simulink model "untitled"  (R2023b)
settings: Solver=VariableStepAuto  StartTime=0.0  StopTime=10  RelTol=1e-3
values from neighbouring files (symbols this model uses):
  A = [0, 1, 0, 0, 0, 0 ... (first row only)    [DESACOPLE.m]    (also in untitled2.m = (subs(A_sym, [qs; fs], [qs0; fs0])))
  B = [0, 0, 0; 50/(25*q3_op^2 +10*q3_op +3), 0, 0;0, 0, 0;0, 2/3, 0;0, 0, 0;0, 0, 2]    [DESACOPLE.m]    (also in untitled2.m = (subs(B_sym, [qs; fs], [qs0; fs0])))
  F = G*P    [DESACOPLE.m]
  G = pinv(E)    [DESACOPLE.m]
  q3_op = 0.2    [DESACOPLE.m]
undefined symbols (not defined in the file or in its folder): A_num, B_num
settings Model: Creator=alejo  LastModifiedBy=alejo

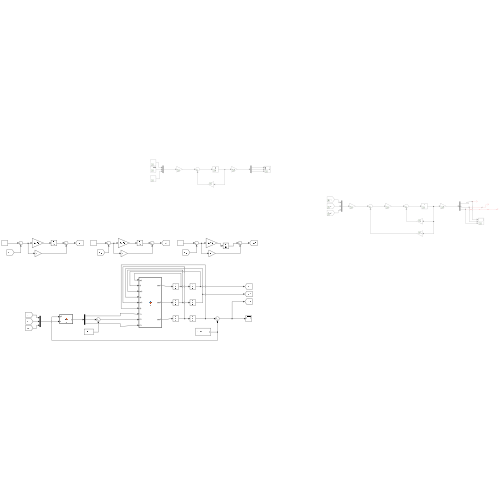
[thumbnail: Simulink's stored preview of the top-level diagram]
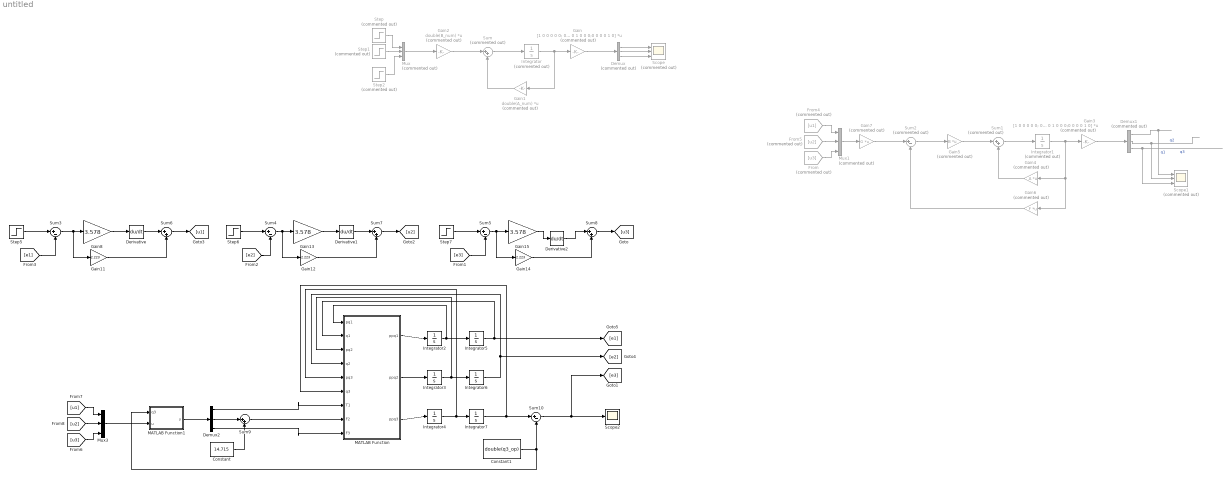
== system untitled ==
  Constant : Constant  Value=14.715
  Constant1 : Constant  Value=double(q3_op)
  Demux : Demux  Commented=on  Outputs=3
  Demux1 : Demux  Commented=on  Outputs=3
  Demux2 : Demux  Outputs=3
  Derivative : Derivative
  Derivative1 : Derivative
  Derivative2 : Derivative
  From : From  Commented=on  GotoTag=u3
  From4 : From  Commented=on  GotoTag=u1
  From5 : From  Commented=on  GotoTag=u2
  Gain : Gain  Commented=on  Gain=[1 0 0 0 0 0; 0 0 1 0 0 0;0 0 0 0 1 0]  Multiplication=Matrix(K*u)
  Gain1 : Gain  Commented=on  Gain=double(A_num)  Multiplication=Matrix(K*u)
  Gain11 : Gain  Gain=2.223
  Gain12 : Gain  Gain=2.223
  Gain13 : Gain  Gain=3.578
  Gain14 : Gain  Gain=2.223
  Gain15 : Gain  Gain=3.578
  Gain2 : Gain  Commented=on  Gain=double(B_num)  Multiplication=Matrix(K*u)
  Gain3 : Gain  Commented=on  Gain=[1 0 0 0 0 0; 0 0 1 0 0 0;0 0 0 0 1 0]  Multiplication=Matrix(K*u)
  Gain4 : Gain  Commented=on  Gain=A  Multiplication=Matrix(K*u)
  Gain5 : Gain  Commented=on  Gain=B  Multiplication=Matrix(K*u)
  Gain6 : Gain  Commented=on  Gain=F  Multiplication=Matrix(K*u)
  Gain7 : Gain  Commented=on  Gain=G  Multiplication=Matrix(K*u)
  Gain8 : Gain  Gain=3.578
  Integrator : Integrator  Commented=on
  Integrator1 : Integrator  Commented=on
  Integrator{2..7} (6 alike) : Integrator
  MATLAB Function : MATLAB Function  TreatAsAtomicUnit=on
  MATLAB Function1 : MATLAB Function  TreatAsAtomicUnit=on
  Mux : Mux  Commented=on  Inputs=3
  Mux1 : Mux  Commented=on  Inputs=3
  Mux3 : Mux  Inputs=3
  Scope : Scope  Commented=on  NumInputPorts=3
  Scope1 : Scope  Commented=on  NumInputPorts=3
  Scope2 : Scope
  Step : Step  Commented=on  SampleTime=0
  Step1 : Step  Commented=on  SampleTime=0
  Step2 : Step  Commented=on  SampleTime=0
  Step5 : Step  Time=0  After=0  SampleTime=0
  Step6 : Step  Time=0  After=0  SampleTime=0
  Step7 : Step  Time=0  SampleTime=0
  Sum : Sum  Commented=on  Inputs=|++
  Sum1 : Sum  Commented=on  Inputs=|++
  Sum{3..5,10} (4 alike) : Sum  Inputs=|+-
  Sum2 : Sum  Commented=on  Inputs=|+-
  Sum{6..9} (4 alike) : Sum  Inputs=|++
  wires:
  Step/1 -> Mux/1
  Step1/1 -> Mux/2
  Mux/1 -> Gain2/1
  Gain2/1 -> Sum/1
  Sum/1 -> Integrator/1
  Integrator/1 -> Gain1/1, Gain/1
  Gain1/1 -> Sum/2
  Gain/1 -> Demux/1
  Demux/2 -> Scope/2
  Demux/1 -> Scope/1
  Step2/1 -> Mux/3
  Demux/3 -> Scope/3
  Demux1/3 -> Scope1/3  "q3"
  Demux1/1 -> Scope1/1  "q1"
  Demux1/2 -> Scope1/2  "q2"
  Gain3/1 -> Demux1/1
  Gain4/1 -> Sum1/2
  Integrator1/1 -> Gain3/1, Gain6/1, Gain4/1
  Sum1/1 -> Integrator1/1
  Gain5/1 -> Sum1/1
  Gain7/1 -> Sum2/1
  Sum2/1 -> Gain5/1
  Gain6/1 -> Sum2/2
  Mux1/1 -> Gain7/1
  Step5/1 -> Sum3/1
  [e1] -> Sum3/2
  From4/1 -> Mux1/1
  [e2] -> Sum4/2
  Step6/1 -> Sum4/1
  Step7/1 -> Sum5/1
  [e3] -> Sum5/2
  From5/1 -> Mux1/2
  From/1 -> Mux1/3
  Gain8/1 -> Derivative/1
  Gain13/1 -> Derivative1/1
  Gain15/1 -> Derivative2/1
  Derivative/1 -> Sum6/1
  Gain11/1 -> Sum6/2
  Sum3/1 -> Gain11/1, Gain8/1
  Sum6/1 -> [u1]
  Derivative1/1 -> Sum7/1
  Derivative2/1 -> Sum8/1
  Gain14/1 -> Sum8/2
  Sum7/1 -> [u2]
  Sum4/1 -> Gain12/1, Gain13/1
  Gain12/1 -> Sum7/2
  Sum5/1 -> Gain14/1, Gain15/1
  Sum8/1 -> [u3]
  MATLAB Function/1(ppq1) -> Integrator2/1
  MATLAB Function/2(ppq2) -> Integrator3/1
  MATLAB Function/3(ppq3) -> Integrator4/1
  Integrator2/1 -> Integrator5/1, MATLAB Function/1(pq1)
  Integrator3/1 -> MATLAB Function/3(pq2), Integrator6/1
  Integrator4/1 -> MATLAB Function/5(pq3), Integrator7/1
  Integrator7/1 -> Sum10/1, MATLAB Function/6(q3)
  MATLAB Function1/1(y) -> Demux2/1
  Demux2/2 -> Sum9/1
  Constant/1 -> Sum9/2
  Demux2/1 -> MATLAB Function/7(T1)
  Demux2/3 -> MATLAB Function/9(F3)
  Sum9/1 -> MATLAB Function/8(F2)
  Constant1/1 -> Sum10/2, MATLAB Function1/1(q3)
  Integrator5/1 -> [e1], MATLAB Function/2(q1)
  [u3] -> Mux3/3
  [u2] -> Mux3/2
  [u1] -> Mux3/1
  Mux3/1 -> MATLAB Function1/2(u)
  Integrator6/1 -> [e2], MATLAB Function/4(q2)
  Sum10/1 -> Scope2/1, [e3]

== matlab function untitled/MATLAB Function1 ==
  data: q3 input; u input; y output
function y = fcn(q3, u)
G = [q3^2/2 + q3/5 + 3/50,   0,   0; 0, 3/2,   0; 0,   0, 1/2];
y = G*u;

== matlab function untitled/MATLAB Function ==
  data: pq1 input; ppq1 output; q1 input; pq2 input; q2 input; pq3 input; q3 input; T1 input; F2 input; F3 input; ppq2 output; ppq3 output
function [ppq1, ppq2, ppq3] = fcn(pq1, q1, pq2, q2, pq3, q3, T1, F2, F3)

ppq1 = (T1-pq1*q3*pq3-pq1*pq3/5)/((q3^2)/2 +q3/5 +3/50);

ppq2 = 2*F2/3 -9.81;

ppq3 = 2*F3 +(pq1^2)*q3 +(pq1^2)/5;
